simulink model "rst_auto_reg_sin_2018a"  (R2018a)
settings: Solver=VariableStepAuto  StartTime=0.0  StopTime=100  RelTol=1e-3
undefined symbols (not defined in the file): A, B, ep, R, S, T, Ta, Tas, tc, Ts, w0
libraries: dspinverses x2
settings Model: Creator=Carlos Henrique  LastModifiedBy=tarci
settings DataIOCC: SaveOutput=off  SaveState=on  SignalLogging=off  DSMLogging=off
settings SFSimCC: SimUseLocalCustomCode=on
settings RTWCC: RTWUseLocalCustomCode=on

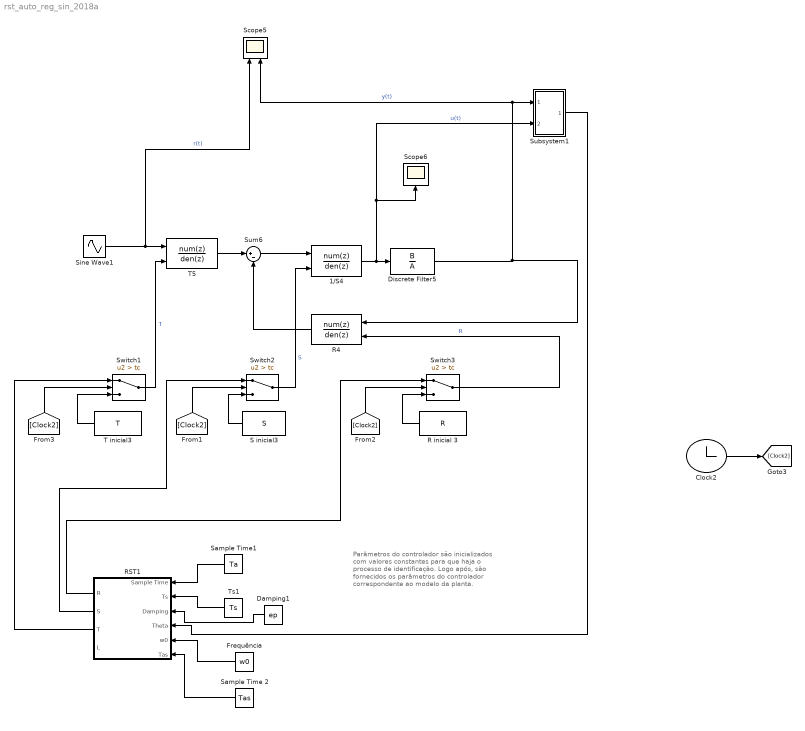
== system rst_auto_reg_sin_2018a ==
  note: Parâmetros do controlador são inicializados
      | com valores constantes para que haja o
      | processo de identificação. Logo após, são
      | fornecidos os parâmetros do controlador
      | correspondente ao modelo da planta.
  1/S4 : DiscreteFilter  Numerator=1  DenominatorSource=Input port  Denominator=1  a0EqualsOne=on
      settings: InputPortMap=u0,p3
  Clock2 : Clock
  Damping1 : Constant  Value=ep
  Discrete Filter5 : DiscreteFilter  Numerator=B  Denominator=A  a0EqualsOne=on
  Frequência : Constant  Value=w0
  R inicial 3 : Constant  Value=R
  R4 : DiscreteFilter  NumeratorSource=Input port  Numerator=[-620.2 131.3]  Denominator=1
      settings: InputPortMap=u0,p1
  RST1 : Subsystem
  S inicial3 : Constant  Value=S
  Sample Time 2 : Constant  Value=Tas
  Sample Time1 : Constant  Value=Ta
  Scope5 : Scope  NumInputPorts=2
  Scope6 : Scope
  Sine Wave1 : Sin  SampleTime=0.1
  Subsystem1 : Subsystem
  Sum6 : Sum  Inputs=|+-
  Switch1 : Switch  Criteria=u2 > Threshold  Threshold=tc
  Switch2 : Switch  Criteria=u2 > Threshold  Threshold=tc
  Switch3 : Switch  Criteria=u2 > Threshold  Threshold=tc
  T inicial3 : Constant  Value=T
  T5 : DiscreteFilter  NumeratorSource=Input port  Numerator=13.39  Denominator=1
      settings: InputPortMap=u0,p1
  Ts1 : Constant  Value=Ts
  wires:
  RST1/1(R) -> Switch3/1
  R4/1 -> Sum6/2
  Sample Time 2/1 -> RST1/6(Tas)
  [Clock2] -> Switch1/2
  Ts1/1 -> RST1/2(Ts)
  S inicial3/1 -> Switch2/3
  RST1/3(T) -> Switch1/1
  T5/1 -> Sum6/1
  Switch3/1 -> R4/2  "R"
  Discrete Filter5/1 -> Scope5/2, Subsystem1/1(y(t)), R4/1  "y(t)"
  Switch2/1 -> 1/S4/2  "S"
  Switch1/1 -> T5/2  "T"
  RST1/2(S) -> Switch2/1
  T inicial3/1 -> Switch1/3
  Sum6/1 -> 1/S4/1
  Sample Time1/1 -> RST1/1(Sample Time)
  Sine Wave1/1 -> T5/1, Scope5/1  "r(t)"
  1/S4/1 -> Discrete Filter5/1, Scope6/1, Subsystem1/2("u(t) ")  "u(t)"
  Damping1/1 -> RST1/3(Damping)
  [Clock2] -> Switch2/2
  Frequência/1 -> RST1/5(w0)
  Subsystem1/1("Theta(t) ") -> RST1/4(Theta)
  [Clock2] -> Switch3/2
  R inicial 3/1 -> Switch3/3
  Clock2/1 -> [Clock2]

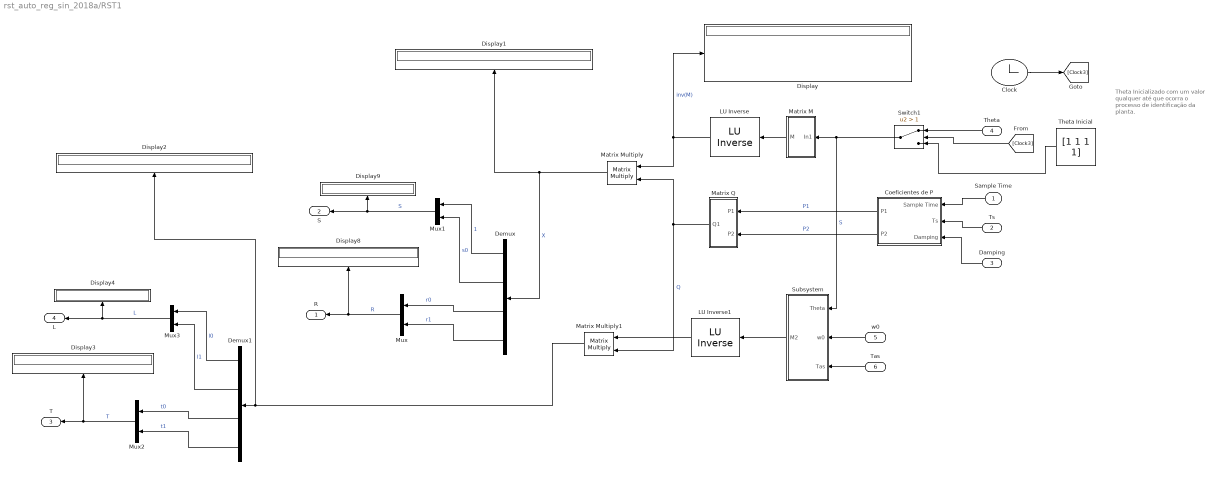
== system rst_auto_reg_sin_2018a/RST1 ==
  note: Theta Inicializado com um
      | valor qualquer até que ocorra
      |  o processo de identificação
      | da planta.
  Sample Time : Inport
  Ts : Inport  Port=2
  Damping : Inport  Port=3
  Theta : Inport  Port=4
  w0 : Inport  Port=5
  Tas : Inport  Port=6
  " LU Inverse" : dspinverses/ LU Inverse
      settings: SourceProductName=DSP System Toolbox
  " LU Inverse1" : dspinverses/ LU Inverse
      settings: SourceProductName=DSP System Toolbox
  Clock : Clock
  Coeficientes de P : Subsystem
  Demux : Demux
  Demux1 : Demux
  Display{,1..4,8..9} (7 alike) : Display
  Matrix M : Subsystem
  Matrix Multiply : Product  Multiplication=Matrix(*)
  Matrix Multiply1 : Product  Multiplication=Matrix(*)
  Matrix Q : Subsystem
  Mux{,1..3} (4 alike) : Mux  Inputs=2
  Subsystem : Subsystem
  Switch1 : Switch  Criteria=u2 > Threshold  Threshold=1
  Theta Inicial : Constant  Value=[1 1 1 1]
  R : Outport
  S : Outport  Port=2
  T : Outport  Port=3
  L : Outport  Port=4
  wires:
  Demux/4 -> Mux/2  "r1"
  Demux/3 -> Mux/1  "r0"
  Demux/2 -> Mux1/2  "s0"
  Demux/1 -> Mux1/1  "1"
  Matrix Q/1(Q1) -> Matrix Multiply1/2, Matrix Multiply/2  "Q"
  Matrix M/1(M) -> " LU Inverse"/1
  Theta Inicial/1 -> Switch1/3
  [Clock3] -> Switch1/2
  Theta/1 -> Switch1/1
  Switch1/1 -> Subsystem/1(Theta), Matrix M/1(In1)  "S"
  Clock/1 -> [Clock3]
  Mux/1 -> Display8/1, R/1  "R"
  Coeficientes de P/1(P1) -> Matrix Q/1(P1)  "P1"
  Sample Time/1 -> Coeficientes de P/1(Sample Time)
  Damping/1 -> Coeficientes de P/3(Damping)
  Ts/1 -> Coeficientes de P/2(Ts)
  Coeficientes de P/2(P2) -> Matrix Q/2(P2)  "P2"
  Mux1/1 -> Display9/1, S/1  "S"
  " LU Inverse"/1 -> Display/1, Matrix Multiply/1  "inv(M)"
  Matrix Multiply/1 -> Display1/1, Demux/1  "X"
  w0/1 -> Subsystem/2(w0)
  Tas/1 -> Subsystem/3(Tas)
  Subsystem/1(M2) -> " LU Inverse1"/1
  " LU Inverse1"/1 -> Matrix Multiply1/1
  Mux3/1 -> L/1, Display4/1  "L"
  Mux2/1 -> T/1, Display3/1  "T"
  Demux1/1 -> Mux3/1  "l0"
  Demux1/2 -> Mux3/2  "l1"
  Demux1/3 -> Mux2/1  "t0"
  Demux1/4 -> Mux2/2  "t1"
  Matrix Multiply1/1 -> Display2/1, Demux1/1

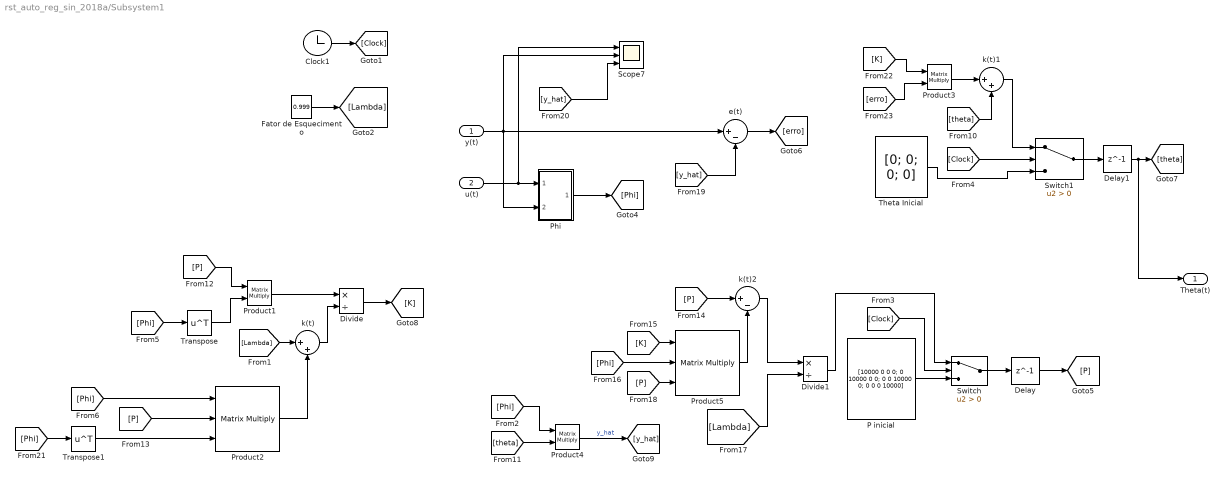
== system rst_auto_reg_sin_2018a/Subsystem1 ==
  y(t) : Inport
  "u(t) " : Inport  Port=2
  Clock1 : Clock
  Delay : Delay  DelayLength=1  InitialCondition=0
  Delay1 : Delay  DelayLength=1  InitialCondition=0
  Divide : Product  Inputs=*/
  Divide1 : Product  Inputs=*/
  "Fator de Esquecimento " : Constant  Value=0.999
  P inicial : Constant  Value=[10000 0 0 0; 0 10000 0 0; 0 0 10000 0; 0 0 0 10000]
  Phi : Subsystem
  Product1 : Product  Multiplication=Matrix(*)
  Product2 : Product  Inputs=3  Multiplication=Matrix(*)
  Product3 : Product  Multiplication=Matrix(*)
  Product4 : Product  Multiplication=Matrix(*)
  Product5 : Product  Inputs=3  Multiplication=Matrix(*)
  Scope7 : Scope  NumInputPorts=3
  Switch : Switch  Criteria=u2 > Threshold
  Switch1 : Switch  Criteria=u2 > Threshold
  "Theta Inicial " : Constant  Value=[0; 0; 0; 0]
  Transpose : Math  Operator=transpose  SaturateOnIntegerOverflow=on
  Transpose1 : Math  Operator=transpose  SaturateOnIntegerOverflow=on
  e(t) : Sum  Inputs=|+-
  k(t) : Sum  Inputs=|++
  k(t)1 : Sum  Inputs=|++
  k(t)2 : Sum  Inputs=|+-
  "Theta(t) " : Outport
  wires:
  Product4/1 -> [y_hat]  "y_hat"
  [Phi] -> Product5/2
  Divide/1 -> [K]
  [Phi] -> Product2/1
  [P] -> Product1/1
  P inicial/1 -> Switch/3
  [K] -> Product5/1
  [y_hat] -> e(t)/2
  [erro] -> Product3/2
  Clock1/1 -> [Clock]
  Transpose/1 -> Product1/2
  [Lambda] -> k(t)/1
  [P] -> Product2/2
  [theta] -> k(t)1/2
  [P] -> k(t)2/1
  [theta] -> Product4/2
  [Clock] -> Switch/2
  [Phi] -> Transpose/1
  Divide1/1 -> Switch/1
  Transpose1/1 -> Product2/3
  "Theta Inicial "/1 -> Switch1/3
  "Fator de Esquecimento "/1 -> [Lambda]
  [P] -> Product5/3
  [Phi] -> Transpose1/1
  Delay/1 -> [P]
  Product3/1 -> k(t)1/1
  e(t)/1 -> [erro]
  Product1/1 -> Divide/1
  [Lambda] -> Divide1/2
  Switch/1 -> Delay/1
  "u(t) "/1 -> Phi/1(u(t)), Scope7/1
  Product5/1 -> k(t)2/2
  Delay1/1 -> [theta], "Theta(t) "/1
  k(t)2/1 -> Divide1/1
  y(t)/1 -> Phi/2(y(t)), Scope7/2, e(t)/1
  [Clock] -> Switch1/2
  Product2/1 -> k(t)/2
  [K] -> Product3/1
  Switch1/1 -> Delay1/1
  [y_hat] -> Scope7/3
  k(t)1/1 -> Switch1/1
  Phi/1(Phi) -> [Phi]
  [Phi] -> Product4/1
  k(t)/1 -> Divide/2

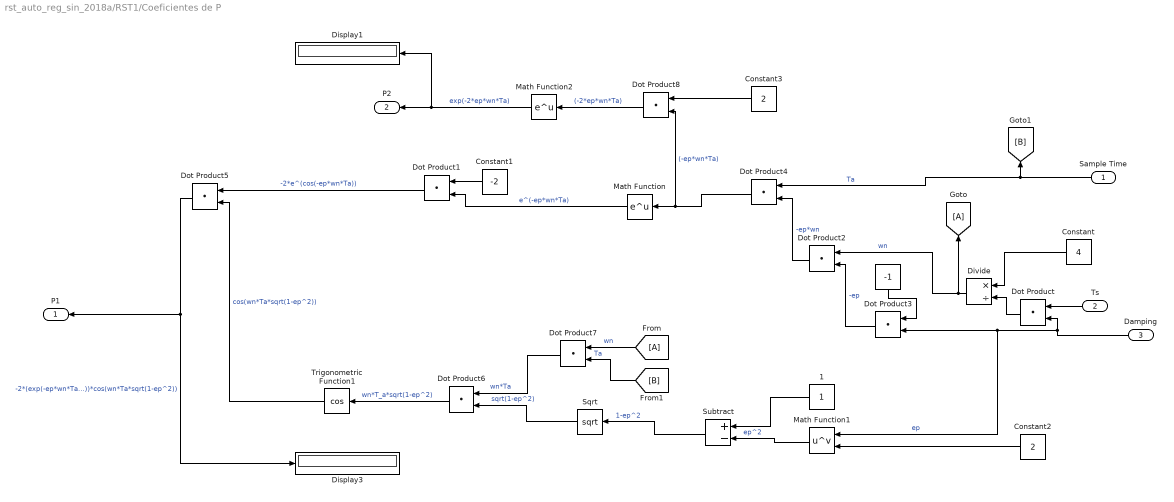
== system rst_auto_reg_sin_2018a/RST1/Coeficientes de P ==
  Sample Time : Inport
  Ts : Inport  Port=2
  Damping : Inport  Port=3
  " " : Constant  Value=-1
  1 : Constant
  Constant : Constant  Value=4
  Constant1 : Constant  Value=-2
  Constant2 : Constant  Value=2
  Constant3 : Constant  Value=2
  Display1 : Display
  Display3 : Display
  Divide : Product  Inputs=*/
  Dot Product{,1..8} (9 alike) : DotProduct  InputSameDT=on  OutDataTypeStr=Inherit: Inherit via internal rule
  Math Function : Math  SaturateOnIntegerOverflow=on
  Math Function1 : Math  Operator=pow  SaturateOnIntegerOverflow=on
  Math Function2 : Math  SaturateOnIntegerOverflow=on
  Sqrt : Sqrt  SaturateOnIntegerOverflow=on
  Subtract : Sum  Inputs=+-
  Trigonometric Function1 : Trigonometry  Operator=cos
  P1 : Outport
  P2 : Outport  Port=2
  wires:
  Math Function2/1 -> P2/1, Display1/1  "exp(-2*ep*wn*Ta)"
  Dot Product8/1 -> Math Function2/1  "(-2*ep*wn*Ta)"
  Constant3/1 -> Dot Product8/1
  Subtract/1 -> Sqrt/1  "1-ep^2"
  Sqrt/1 -> Dot Product6/2  "sqrt(1-ep^2)"
  Dot Product4/1 -> Math Function/1, Dot Product8/2  "(-ep*wn*Ta)"
  Dot Product6/1 -> Trigonometric Function1/1  "wn*T_a*sqrt(1-ep^2)"
  [B] -> Dot Product7/2  "Ta"
  Dot Product2/1 -> Dot Product4/2  "-ep*wn"
  Constant1/1 -> Dot Product1/1
  1/1 -> Subtract/1
  Constant2/1 -> Math Function1/2
  Dot Product1/1 -> Dot Product5/1  "-2*e^(cos(-ep*wn*Ta))"
  Math Function1/1 -> Subtract/2  "ep^2"
  Sample Time/1 -> [B], Dot Product4/1  "Ta"
  Dot Product7/1 -> Dot Product6/1  "wn*Ta"
  Constant/1 -> Divide/1
  Damping/1 -> Dot Product/2, Dot Product3/2, Math Function1/1  "ep"
  Dot Product3/1 -> Dot Product2/2  "-ep"
  Dot Product/1 -> Divide/2
  Ts/1 -> Dot Product/1
  Trigonometric Function1/1 -> Dot Product5/2  "cos(wn*Ta*sqrt(1-ep^2))"
  Dot Product5/1 -> Display3/1, P1/1  "-2*(exp(-ep*wn*Ta))*cos(wn*Ta*sqrt(1-ep^2))"
  " "/1 -> Dot Product3/1
  [A] -> Dot Product7/1  "wn"
  Divide/1 -> Dot Product2/1, [A]  "wn"
  Math Function/1 -> Dot Product1/2  "e^(-ep*wn*Ta)"

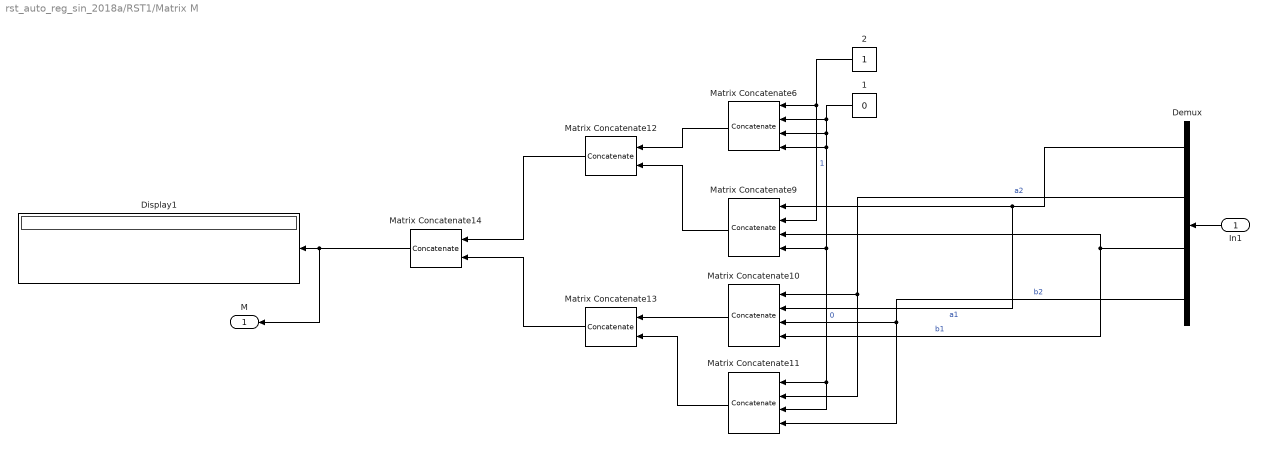
== system rst_auto_reg_sin_2018a/RST1/Matrix M ==
  In1 : Inport
  " 1" : Constant  Value=0
  2 : Constant
  Demux : Demux
  Display1 : Display
  Matrix Concatenate{6,9..11} (4 alike) : Concatenate  NumInputs=4  Mode=Multidimensional array  ConcatenateDimension=2
  Matrix Concatenate12 : Concatenate  Mode=Multidimensional array
  Matrix Concatenate13 : Concatenate  Mode=Multidimensional array
  Matrix Concatenate14 : Concatenate  Mode=Multidimensional array
  M : Outport
  wires:
  Matrix Concatenate12/1 -> Matrix Concatenate14/1
  Matrix Concatenate13/1 -> Matrix Concatenate14/2
  Matrix Concatenate11/1 -> Matrix Concatenate13/2
  Matrix Concatenate10/1 -> Matrix Concatenate13/1
  Matrix Concatenate9/1 -> Matrix Concatenate12/2
  Matrix Concatenate6/1 -> Matrix Concatenate12/1
  " 1"/1 -> Matrix Concatenate6/2, Matrix Concatenate6/4, Matrix Concatenate9/4, Matrix Concatenate11/1, Matrix Concatenate11/3, Matrix Concatenate6/3  "0"
  2/1 -> Matrix Concatenate6/1, Matrix Concatenate9/2  "1"
  Demux/2 -> Matrix Concatenate10/1, Matrix Concatenate11/2  "a2"
  Demux/4 -> Matrix Concatenate10/3, Matrix Concatenate11/4  "b2"
  Demux/1 -> Matrix Concatenate9/1, Matrix Concatenate10/2  "a1"
  Matrix Concatenate14/1 -> Display1/1, M/1
  Demux/3 -> Matrix Concatenate10/4, Matrix Concatenate9/3  "b1"
  In1/1 -> Demux/1

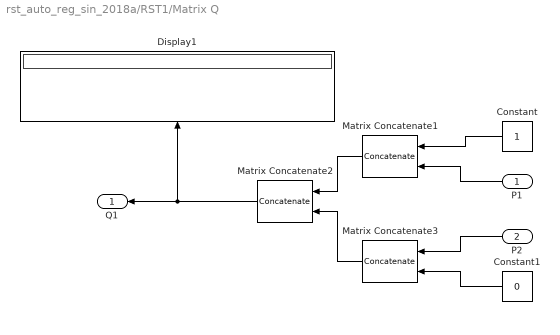
== system rst_auto_reg_sin_2018a/RST1/Matrix Q ==
  P1 : Inport
  P2 : Inport  Port=2
  Constant : Constant
  Constant1 : Constant  Value=0
  Display1 : Display
  Matrix Concatenate1 : Concatenate  Mode=Multidimensional array
  Matrix Concatenate2 : Concatenate  Mode=Multidimensional array
  Matrix Concatenate3 : Concatenate  Mode=Multidimensional array
  Q1 : Outport
  wires:
  Constant1/1 -> Matrix Concatenate3/2
  Constant/1 -> Matrix Concatenate1/1
  P1/1 -> Matrix Concatenate1/2
  P2/1 -> Matrix Concatenate3/1
  Matrix Concatenate3/1 -> Matrix Concatenate2/2
  Matrix Concatenate2/1 -> Display1/1, Q1/1
  Matrix Concatenate1/1 -> Matrix Concatenate2/1

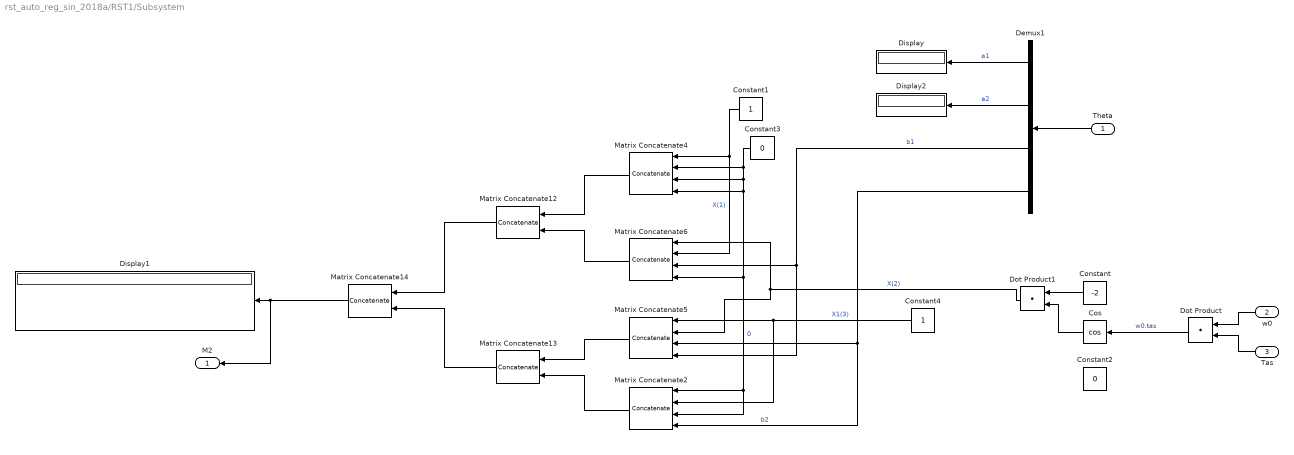
== system rst_auto_reg_sin_2018a/RST1/Subsystem ==
  Theta : Inport
  w0 : Inport  Port=2
  Tas : Inport  Port=3
  Constant : Constant  Value=-2
  Constant1 : Constant
  Constant2 : Constant  Value=0
  Constant3 : Constant  Value=0
  Constant4 : Constant
  Cos : Trigonometry  Operator=cos
  Demux1 : Demux
  Display : Display
  Display1 : Display
  Display2 : Display
  Dot Product : DotProduct  InputSameDT=on  OutDataTypeStr=Inherit: Inherit via internal rule
  Dot Product1 : DotProduct  InputSameDT=on  OutDataTypeStr=Inherit: Inherit via internal rule
  Matrix Concatenate12 : Concatenate  Mode=Multidimensional array
  Matrix Concatenate13 : Concatenate  Mode=Multidimensional array
  Matrix Concatenate14 : Concatenate  Mode=Multidimensional array
  Matrix Concatenate{2,4..6} (4 alike) : Concatenate  NumInputs=4  Mode=Multidimensional array  ConcatenateDimension=2
  M2 : Outport
  wires:
  Constant/1 -> Dot Product1/1
  Cos/1 -> Dot Product1/2
  Matrix Concatenate6/1 -> Matrix Concatenate12/2
  Demux1/2 -> Display2/1  "a2"
  Dot Product/1 -> Cos/1  "w0.tas"
  Tas/1 -> Dot Product/2
  w0/1 -> Dot Product/1
  Theta/1 -> Demux1/1
  Demux1/1 -> Display/1  "a1"
  Constant1/1 -> Matrix Concatenate6/2, Matrix Concatenate4/1  "X(1)"
  Constant3/1 -> Matrix Concatenate4/3, Matrix Concatenate2/3, Matrix Concatenate2/1, Matrix Concatenate6/4, Matrix Concatenate4/4, Matrix Concatenate4/2  "0"
  Dot Product1/1 -> Matrix Concatenate5/2, Matrix Concatenate6/1  "X(2)"
  Constant4/1 -> Matrix Concatenate2/2, Matrix Concatenate5/1  "X1(3)"
  Demux1/3 -> Matrix Concatenate5/4, Matrix Concatenate6/3  "b1"
  Demux1/4 -> Matrix Concatenate2/4, Matrix Concatenate5/3  "b2"
  Matrix Concatenate14/1 -> Display1/1, M2/1
  Matrix Concatenate13/1 -> Matrix Concatenate14/2
  Matrix Concatenate12/1 -> Matrix Concatenate14/1
  Matrix Concatenate4/1 -> Matrix Concatenate12/1
  Matrix Concatenate5/1 -> Matrix Concatenate13/1
  Matrix Concatenate2/1 -> Matrix Concatenate13/2

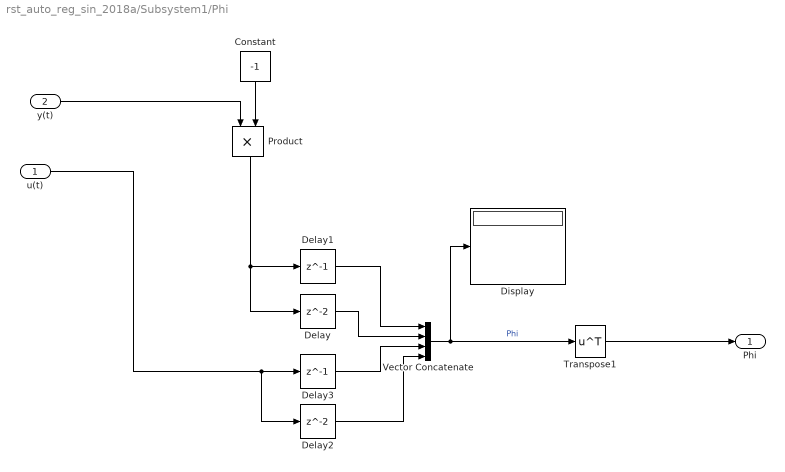
== system rst_auto_reg_sin_2018a/Subsystem1/Phi ==
  u(t) : Inport
  y(t) : Inport  Port=2
  Constant : Constant  Value=-1
  Delay : Delay
  Delay1 : Delay  DelayLength=1
  Delay2 : Delay
  Delay3 : Delay  DelayLength=1
  Display : Display
  Product : Product
  Transpose1 : Math  Operator=transpose  SaturateOnIntegerOverflow=on
  Vector Concatenate : Concatenate  NumInputs=4
  Phi : Outport
  wires:
  Product/1 -> Delay1/1, Delay/1
  Constant/1 -> Product/2
  Transpose1/1 -> Phi/1
  Delay1/1 -> Vector Concatenate/1
  Delay2/1 -> Vector Concatenate/4
  Delay3/1 -> Vector Concatenate/3
  y(t)/1 -> Product/1
  Delay/1 -> Vector Concatenate/2
  Vector Concatenate/1 -> Display/1, Transpose1/1  "Phi"
  u(t)/1 -> Delay3/1, Delay2/1
